simulink model "case_study_3"  (R2013a)
settings: Solver=ode45  SolverMode=SingleTasking  StartTime=0.0  StopTime=0.1  FixedStep=0.0001  RelTol=1e-2
undefined symbols (not defined in the file): f, ids, iqs, is, Ld, LL, Lq, P, RL, Rs, w
libraries: powerlib x34, simulink x12
settings Model: Creator=Asim Khan  LastModifiedBy=Sony
settings DataIOCC: SignalLoggingSaveFormat=ModelDataLogs
settings OptimizationCC: BlockReduction=off  BooleanDataType=off
settings DebuggingCC: SaveWithParameterizedLinksMsg=none  SignalResolutionControl=TryResolveAllWithWarning  SolverPrmCheckMsg=none  MultiTaskDSMMsg=warning  MultiTaskCondExecSysMsg=none  StrictBusMsg=None
settings HardwareCC: TargetUnknown=on
settings RTWCC: IncludeERTFirstTime=on

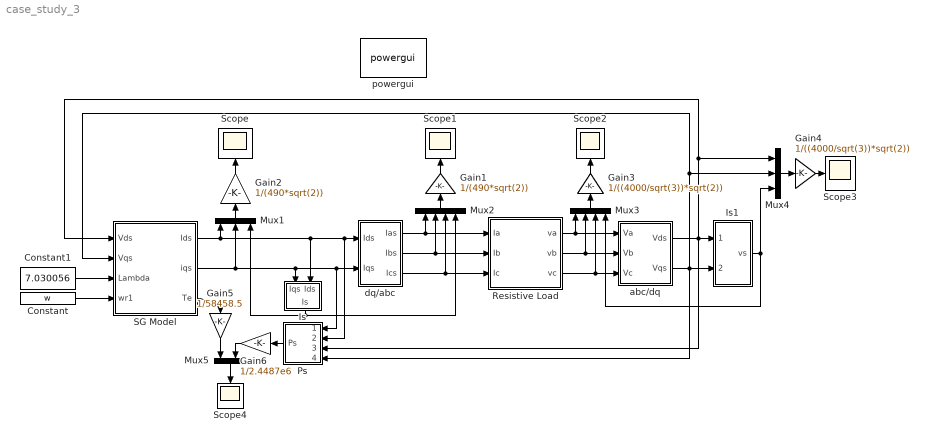
== system case_study_3 ==
  Constant : Constant  Value=w
  Constant1 : Constant  Value=7.030056
  Gain1 : Gain  Gain=1/(490*sqrt(2))
  Gain2 : Gain  Gain=1/(490*sqrt(2))
  Gain3 : Gain  Gain=1/((4000/sqrt(3))*sqrt(2))
  Gain4 : Gain  Gain=1/((4000/sqrt(3))*sqrt(2))
  Gain5 : Gain  Gain=1/58458.5
  Gain6 : Gain  Gain=1/2.4487e6
  Is : Subsystem
  Is1 : Subsystem
  Mux1 : Mux  Inputs=3
  Mux2 : Mux
  Mux3 : Mux
  Mux4 : Mux  Inputs=3
  Mux5 : Mux  Inputs=2
  Ps : Subsystem
  Resistive Load : Subsystem
  SG Model : Subsystem
  Scope{,1..4} (5 alike) : Scope
      Scope settings: YMin=0  YMax=1
      Scope1 settings: YMin=-0.8  YMax=0.8
      Scope4 settings: YMin=-20  YMax=20
  abc/dq : Subsystem
  "dq/abc " : Subsystem
  powergui : powerlib/powergui  Priority=1  SimulationMode=Continuous  SolverType=Tustin  SampleTime=50e-6  frequency=60  SPID=on  DisableSnubberDevices=off  DisableRonSwitches=on  DisableVfSwitches=on  SwTol=0  Interpol=off  DisplayEquations=off  frequencyindice=0  Pbase=100e6  ErrMax=1e-4  Iterations=50  UnitsV=kV  UnitsW=MW  FunctionMessages=off  echomessages=off  HookPort=off  EnableUseOfTLC=off  x0status=steady  RestoreLinks=warning  ResistiveCurrentMeasurement=off  Frange=[0:2:500]  Ylog=off  Xlog=on  ShowGrid=off  save=off  variable=ZData  ZoomFFT=off  StartTime=0.0  cycles=1  DisplayStyle=1  fundamental=60  FreqAxis=off  MaxFrequency=1000  frequencyindicesteady=1  RmsSteady=1  display=off  Ts=0  methode=off
  wires:
  SG Model/2(iqs) -> "dq/abc "/2(Iqs), Ps/1(Iqs), Is/1(Iqs), Mux1/2
  Resistive Load/1(va) -> abc/dq/1(Va), Mux3/1
  Resistive Load/2(vb) -> Mux3/2, abc/dq/2(Vb)
  Resistive Load/3(vc) -> abc/dq/3(Vc), Mux3/3
  Constant1/1 -> SG Model/3(Lambda)
  "dq/abc "/1(Ias) -> Resistive Load/1(Ia), Mux2/1
  "dq/abc "/2(Ibs) -> Resistive Load/2(Ib), Mux2/2
  "dq/abc "/3("Ics ") -> Resistive Load/3(Ic), Mux2/3
  abc/dq/1(Vds) -> Ps/3(vds), SG Model/1(Vds), Mux4/1, Is1/1(vds)
  SG Model/1(Ids) -> "dq/abc "/1(Ids), Ps/2(Ids), Is/2(Ids), Mux1/1
  Constant/1 -> SG Model/4(wr1)
  Mux5/1 -> Scope4/1
  Mux1/1 -> Gain2/1
  Gain2/1 -> Scope/1
  Mux2/1 -> Gain1/1
  Gain1/1 -> Scope1/1
  Mux3/1 -> Gain3/1
  Gain3/1 -> Scope2/1
  Mux4/1 -> Gain4/1
  Gain4/1 -> Scope3/1
  Is/1(Is) -> Mux2/4, Mux1/3
  abc/dq/2(Vqs) -> Ps/4(vqs), Is1/2(vqs), SG Model/2(Vqs), Mux4/2
  SG Model/3(Te) -> Gain5/1
  Gain5/1 -> Mux5/1
  Ps/1(Ps) -> Gain6/1
  Gain6/1 -> Mux5/2
  Is1/1(vs) -> Mux3/4, Mux4/3

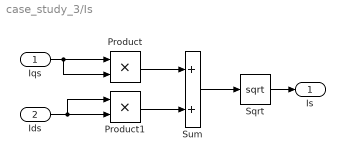
== system case_study_3/Is ==
  Iqs : Inport
  Ids : Inport  Port=2
  Product : Product
  Product1 : Product
  Sqrt : Sqrt  SaturateOnIntegerOverflow=on
  Sum : Sum
  Is : Outport
  wires:
  Iqs/1 -> Product/2, Product/1
  Ids/1 -> Product1/2, Product1/1
  Product/1 -> Sum/1
  Product1/1 -> Sum/2
  Sum/1 -> Sqrt/1
  Sqrt/1 -> Is/1

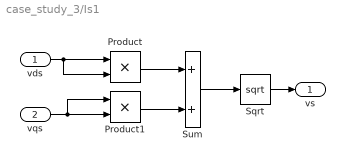
== system case_study_3/Is1 ==
  vds : Inport
  vqs : Inport  Port=2
  Product : Product
  Product1 : Product
  Sqrt : Sqrt  SaturateOnIntegerOverflow=on
  Sum : Sum
  vs : Outport
  wires:
  vds/1 -> Product/2, Product/1
  vqs/1 -> Product1/2, Product1/1
  Product/1 -> Sum/1
  Product1/1 -> Sum/2
  Sum/1 -> Sqrt/1
  Sqrt/1 -> vs/1

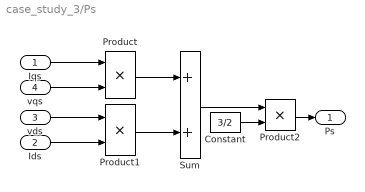
== system case_study_3/Ps ==
  Iqs : Inport
  Ids : Inport  Port=2
  vds : Inport  Port=3
  vqs : Inport  Port=4
  Constant : Constant  Value=3/2
  Product : Product
  Product1 : Product
  Product2 : Product
  Sum : Sum
  Ps : Outport
  wires:
  Iqs/1 -> Product/1
  Ids/1 -> Product1/2
  Product/1 -> Sum/1
  Product1/1 -> Sum/2
  Sum/1 -> Product2/1
  Constant/1 -> Product2/2
  vqs/1 -> Product/2
  vds/1 -> Product1/1
  Product2/1 -> Ps/1

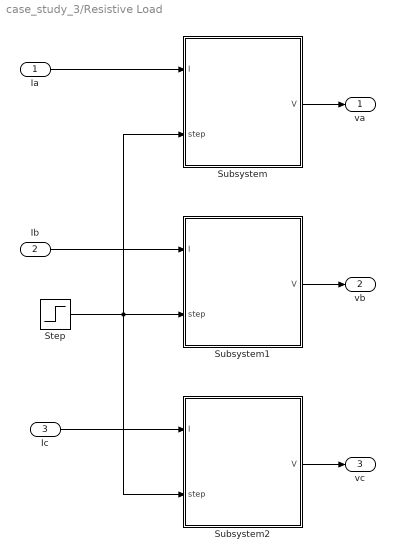
== system case_study_3/Resistive Load ==
  Ia : Inport
  Ib : Inport  Port=2
  Ic : Inport  Port=3
  Step : Step  Time=0.05  SampleTime=0
  Subsystem : Subsystem
  Subsystem1 : Subsystem
  Subsystem2 : Subsystem
  va : Outport
  vb : Outport  Port=2
  vc : Outport  Port=3
  wires:
  Step/1 -> Subsystem2/2(step), Subsystem1/2(step), Subsystem/2(step)
  Ia/1 -> Subsystem/1(I)
  Subsystem/1(V) -> va/1
  Subsystem1/1(V) -> vb/1
  Ib/1 -> Subsystem1/1(I)
  Ic/1 -> Subsystem2/1(I)
  Subsystem2/1(V) -> vc/1

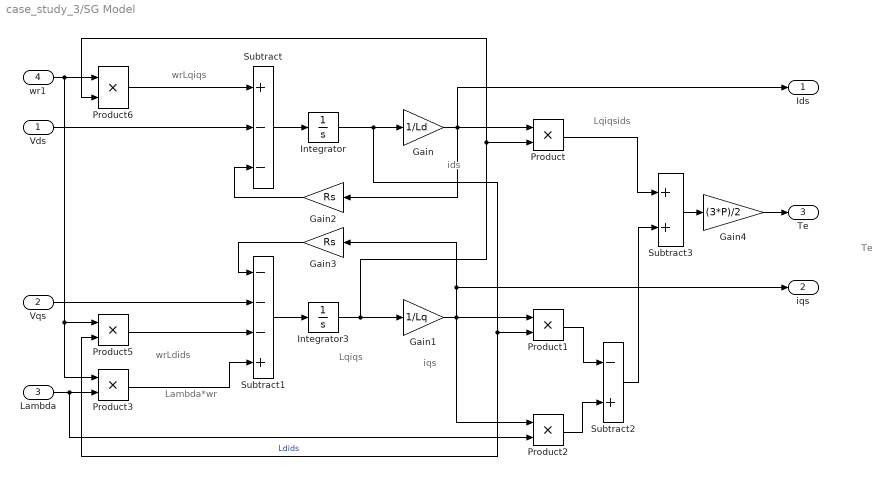
== system case_study_3/SG Model ==
  note: Lqiqsids
  note: iqs
  note: Te
  note: Lqiqs
  note: wrLqiqs
  note: wrLdids
  note: Lambda*wr
  note: ids
  Vds : Inport
  Vqs : Inport  Port=2
  Lambda : Inport  Port=3
  wr1 : Inport  Port=4
  Gain : Gain  Gain=1/Ld
  Gain1 : Gain  Gain=1/Lq
  Gain2 : Gain  Gain=Rs
  Gain3 : Gain  Gain=Rs
  Gain4 : Gain  Gain=(3*P)/2
  Integrator : Integrator  InitialCondition=ids*Ld
  Integrator3 : Integrator  InitialCondition=iqs*Lq
  Product{,1..3,5..6} (6 alike) : Product
  Subtract : Sum  Inputs=+--
  Subtract1 : Sum  Inputs=---+
  Subtract2 : Sum  Inputs=-+
  Subtract3 : Sum
  Ids : Outport
  iqs : Outport  Port=2
  Te : Outport  Port=3
  wires:
  Subtract/1 -> Integrator/1
  Subtract1/1 -> Integrator3/1
  Subtract3/1 -> Gain4/1
  Gain2/1 -> Subtract/3
  Gain3/1 -> Subtract1/1
  Integrator/1 -> Product1/2, Product5/2, Gain/1  "Ldids"
  Gain/1 -> Gain2/1, Product/1, Ids/1
  Gain1/1 -> Gain3/1, iqs/1, Product1/1, Product2/1
  Lambda/1 -> Product2/2, Product3/2
  Product/1 -> Subtract3/1
  Product1/1 -> Subtract2/1
  Product2/1 -> Subtract2/2
  Subtract2/1 -> Subtract3/2
  Gain4/1 -> Te/1
  Integrator3/1 -> Product6/2, Product/2, Gain1/1
  Vqs/1 -> Subtract1/2
  Vds/1 -> Subtract/2
  wr1/1 -> Product6/1, Product5/1, Product3/1
  Product6/1 -> Subtract/1
  Product5/1 -> Subtract1/3
  Product3/1 -> Subtract1/4

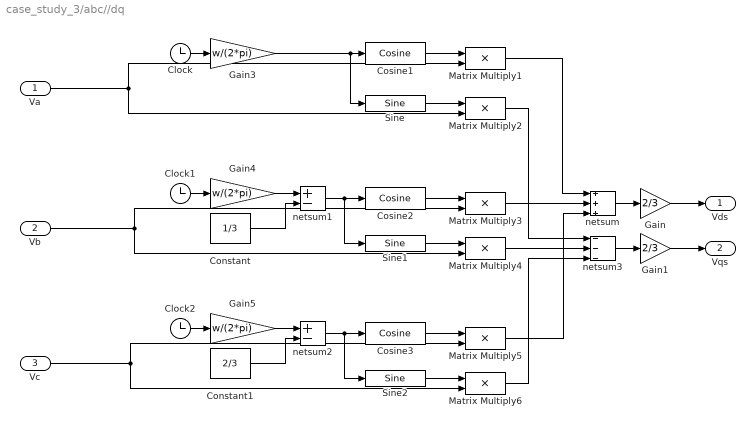
== system case_study_3/abc//dq ==
  Va : Inport
  Vb : Inport  Port=2
  Vc : Inport  Port=3
  Clock : Clock
  Clock1 : Clock
  Clock2 : Clock
  Constant : Constant  Value=1/3
  Constant1 : Constant  Value=2/3
  Cosine1 : simulink/Lookup Tables/Cosine  Formula=cos(2*pi*u)  NumDataPoints=(2^5)+1  OutputWordLength=16
  Cosine2 : simulink/Lookup Tables/Cosine  Formula=cos(2*pi*u)  NumDataPoints=(2^5)+1  OutputWordLength=16
  Cosine3 : simulink/Lookup Tables/Cosine  Formula=cos(2*pi*u)  NumDataPoints=(2^5)+1  OutputWordLength=16
  Gain : Gain  Gain=2/3
  Gain1 : Gain  Gain=2/3
  Gain3 : Gain  Gain=w/(2*pi)
  Gain4 : Gain  Gain=w/(2*pi)
  Gain5 : Gain  Gain=w/(2*pi)
  Matrix Multiply{1..6} (6 alike) : Product
  Sine : simulink/Lookup Tables/Sine  Formula=sin(2*pi*u)  NumDataPoints=(2^5)+1  OutputWordLength=16
  Sine1 : simulink/Lookup Tables/Sine  Formula=sin(2*pi*u)  NumDataPoints=(2^5)+1  OutputWordLength=16
  Sine2 : simulink/Lookup Tables/Sine  Formula=sin(2*pi*u)  NumDataPoints=(2^5)+1  OutputWordLength=16
  netsum : Sum  Inputs=+++  SaturateOnIntegerOverflow=on  InputSameDT=on  OutDataTypeStr=Inherit: Same as first input
  netsum1 : Sum  Inputs=+-  SaturateOnIntegerOverflow=on  InputSameDT=on  OutDataTypeStr=Inherit: Same as first input
  netsum2 : Sum  Inputs=+-  SaturateOnIntegerOverflow=on  InputSameDT=on  OutDataTypeStr=Inherit: Same as first input
  netsum3 : Sum  Inputs=---  SaturateOnIntegerOverflow=on  InputSameDT=on  OutDataTypeStr=Inherit: Same as first input
  Vds : Outport
  Vqs : Outport  Port=2
  wires:
  Cosine1/1 -> Matrix Multiply1/1
  Clock/1 -> Gain3/1
  Gain3/1 -> Sine/1, Cosine1/1
  Sine/1 -> Matrix Multiply2/1
  Cosine2/1 -> Matrix Multiply3/1
  Clock1/1 -> Gain4/1
  Sine1/1 -> Matrix Multiply4/1
  Gain4/1 -> netsum1/1
  netsum1/1 -> Sine1/1, Cosine2/1
  Constant/1 -> netsum1/2
  Cosine3/1 -> Matrix Multiply5/1
  Clock2/1 -> Gain5/1
  Sine2/1 -> Matrix Multiply6/1
  Gain5/1 -> netsum2/1
  netsum2/1 -> Sine2/1, Cosine3/1
  Constant1/1 -> netsum2/2
  Gain1/1 -> Vqs/1
  Gain/1 -> Vds/1
  Va/1 -> Matrix Multiply2/2, Matrix Multiply1/2
  Vb/1 -> Matrix Multiply4/2, Matrix Multiply3/2
  Vc/1 -> Matrix Multiply6/2, Matrix Multiply5/2
  Matrix Multiply1/1 -> netsum/1
  Matrix Multiply3/1 -> netsum/2
  Matrix Multiply5/1 -> netsum/3
  netsum/1 -> Gain/1
  netsum3/1 -> Gain1/1
  Matrix Multiply2/1 -> netsum3/1
  Matrix Multiply4/1 -> netsum3/2
  Matrix Multiply6/1 -> netsum3/3

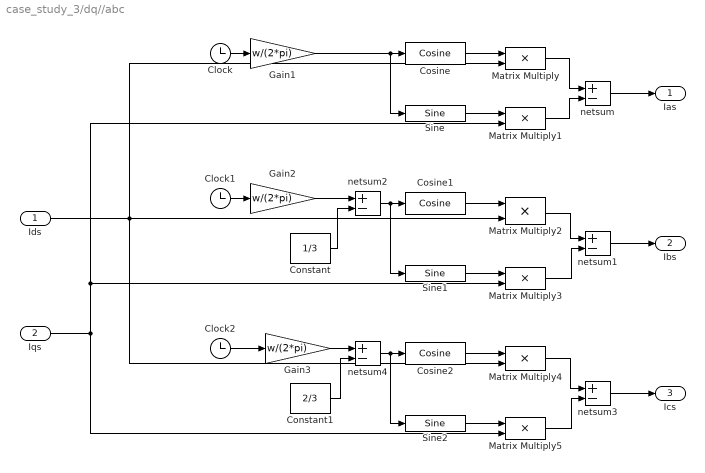
== system case_study_3/dq//abc  ==
  Ids : Inport
  Iqs : Inport  Port=2
  Clock : Clock
  Clock1 : Clock
  Clock2 : Clock
  Constant : Constant  Value=1/3
  Constant1 : Constant  Value=2/3
  Cosine : simulink/Lookup Tables/Cosine  Formula=cos(2*pi*u)  NumDataPoints=(2^5)+1  OutputWordLength=16
  Cosine1 : simulink/Lookup Tables/Cosine  Formula=cos(2*pi*u)  NumDataPoints=(2^5)+1  OutputWordLength=16
  Cosine2 : simulink/Lookup Tables/Cosine  Formula=cos(2*pi*u)  NumDataPoints=(2^5)+1  OutputWordLength=16
  Gain1 : Gain  Gain=w/(2*pi)
  Gain2 : Gain  Gain=w/(2*pi)
  Gain3 : Gain  Gain=w/(2*pi)
  Matrix Multiply{,1..5} (6 alike) : Product
  Sine : simulink/Lookup Tables/Sine  Formula=sin(2*pi*u)  NumDataPoints=(2^5)+1  OutputWordLength=16
  Sine1 : simulink/Lookup Tables/Sine  Formula=sin(2*pi*u)  NumDataPoints=(2^5)+1  OutputWordLength=16
  Sine2 : simulink/Lookup Tables/Sine  Formula=sin(2*pi*u)  NumDataPoints=(2^5)+1  OutputWordLength=16
  netsum{,1..4} (5 alike) : Sum  Inputs=+-  SaturateOnIntegerOverflow=on  InputSameDT=on  OutDataTypeStr=Inherit: Same as first input
  Ias : Outport
  Ibs : Outport  Port=2
  "Ics " : Outport  Port=3
  wires:
  Clock/1 -> Gain1/1
  Gain1/1 -> Sine/1, Cosine/1
  Matrix Multiply/1 -> netsum/1
  Matrix Multiply1/1 -> netsum/2
  netsum/1 -> Ias/1
  Clock1/1 -> Gain2/1
  Sine1/1 -> Matrix Multiply3/1
  Matrix Multiply2/1 -> netsum1/1
  Matrix Multiply3/1 -> netsum1/2
  netsum1/1 -> Ibs/1
  Gain2/1 -> netsum2/1
  netsum2/1 -> Sine1/1, Cosine1/1
  Constant/1 -> netsum2/2
  Clock2/1 -> Gain3/1
  Sine2/1 -> Matrix Multiply5/1
  Matrix Multiply4/1 -> netsum3/1
  Matrix Multiply5/1 -> netsum3/2
  netsum3/1 -> "Ics "/1
  Gain3/1 -> netsum4/1
  netsum4/1 -> Sine2/1, Cosine2/1
  Constant1/1 -> netsum4/2
  Ids/1 -> Matrix Multiply4/2, Matrix Multiply/2, Matrix Multiply2/2
  Iqs/1 -> Matrix Multiply1/2, Matrix Multiply3/2, Matrix Multiply5/2
  Cosine/1 -> Matrix Multiply/1
  Sine/1 -> Matrix Multiply1/1
  Cosine1/1 -> Matrix Multiply2/1
  Cosine2/1 -> Matrix Multiply4/1

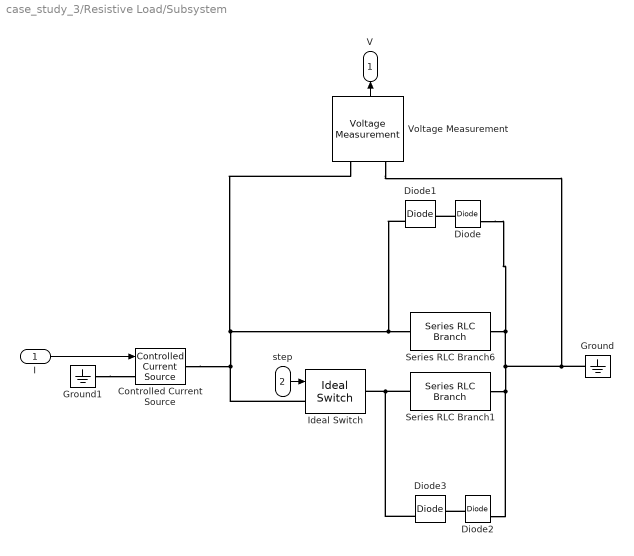
== system case_study_3/Resistive Load/Subsystem ==
  I : Inport
  step : Inport  Port=2
  Controlled Current Source : powerlib/Electrical Sources/Controlled Current Source  Initialize=off  Source_Type=AC  Amplitude=is  Phase=90  Frequency=f  Measurements=None
  Diode{,1..3} (4 alike) : powerlib/Power Electronics/Diode  Ron=0.001  Lon=0  Vf=0.8  IC=0  UseSnubber=off  Rs=Rsnubber  Cs=inf  Measurements=on
  Ground : powerlib/Elements/Ground  LConnTagsString=a
  Ground1 : powerlib/Elements/Ground  LConnTagsString=a
  Ideal Switch : powerlib/Power Electronics/Ideal Switch  Ron=0.001  Lon=0  IC=0  Rs=inf  Cs=inf  Measurements=off
  Series RLC Branch1 : powerlib/Elements/Series RLC Branch  LConnTagsString=__new0  RConnTagsString=__new0  BranchType=RL  Resistance=RL  Inductance=LL  SetiL0=on  InitialCurrent=is  Capacitance=0  Setx0=off  InitialVoltage=0  Measurements=None
  Series RLC Branch6 : powerlib/Elements/Series RLC Branch  LConnTagsString=__new0  RConnTagsString=__new0  BranchType=RL  Resistance=RL  Inductance=LL  SetiL0=on  InitialCurrent=is  Capacitance=0  Setx0=off  InitialVoltage=0  Measurements=None
  Voltage Measurement : powerlib/Measurements/Voltage Measurement  PhasorSimulation=off  OutputType=Complex  PSBequivalent=0
  V : Outport
  wires:
  Voltage Measurement/1 -> V/1
  I/1 -> Controlled Current Source/1
  step/1 -> Ideal Switch/1
  connections:
  Series RLC Branch1/LConn1 -- Diode3/RConn1 -- Ideal Switch/RConn1
  Controlled Current Source/RConn1 -- Ideal Switch/LConn1 -- Voltage Measurement/LConn1 -- Diode1/RConn1 -- Series RLC Branch6/LConn1
  Voltage Measurement/LConn2 -- Ground/LConn1 -- Diode/RConn1 -- Series RLC Branch6/RConn1 -- Diode2/RConn1 -- Series RLC Branch1/RConn1
  Ground1/LConn1 -- Controlled Current Source/LConn1
  Diode/LConn1 -- Diode1/LConn1
  Diode2/LConn1 -- Diode3/LConn1

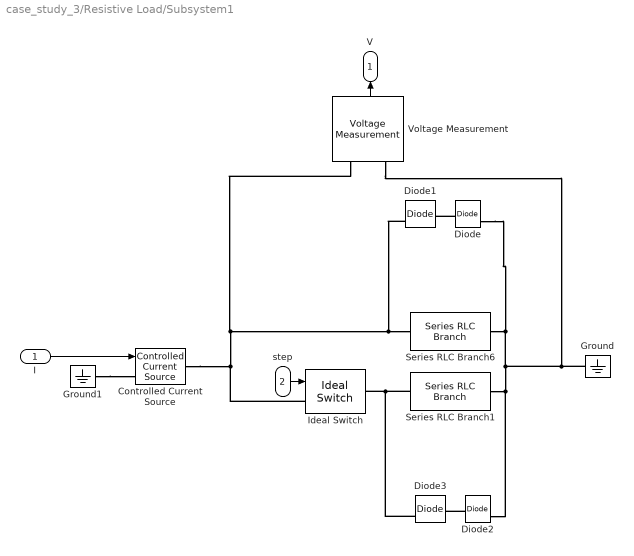
== system case_study_3/Resistive Load/Subsystem1 ==
  I : Inport
  step : Inport  Port=2
  Controlled Current Source : powerlib/Electrical Sources/Controlled Current Source  Initialize=off  Source_Type=AC  Amplitude=is  Phase=90  Frequency=f  Measurements=None
  Diode{,1..3} (4 alike) : powerlib/Power Electronics/Diode  Ron=0.001  Lon=0  Vf=0.8  IC=0  UseSnubber=off  Rs=Rsnubber  Cs=inf  Measurements=on
  Ground : powerlib/Elements/Ground  LConnTagsString=a
  Ground1 : powerlib/Elements/Ground  LConnTagsString=a
  Ideal Switch : powerlib/Power Electronics/Ideal Switch  Ron=0.001  Lon=0  IC=0  Rs=inf  Cs=inf  Measurements=off
  Series RLC Branch1 : powerlib/Elements/Series RLC Branch  LConnTagsString=__new0  RConnTagsString=__new0  BranchType=RL  Resistance=RL  Inductance=LL  SetiL0=on  InitialCurrent=is  Capacitance=0  Setx0=off  InitialVoltage=0  Measurements=None
  Series RLC Branch6 : powerlib/Elements/Series RLC Branch  LConnTagsString=__new0  RConnTagsString=__new0  BranchType=RL  Resistance=RL  Inductance=LL  SetiL0=on  InitialCurrent=is  Capacitance=0  Setx0=off  InitialVoltage=0  Measurements=None
  Voltage Measurement : powerlib/Measurements/Voltage Measurement  PhasorSimulation=off  OutputType=Complex  PSBequivalent=0
  V : Outport
  wires:
  Voltage Measurement/1 -> V/1
  I/1 -> Controlled Current Source/1
  step/1 -> Ideal Switch/1
  connections:
  Diode3/RConn1 -- Series RLC Branch1/LConn1 -- Ideal Switch/RConn1
  Diode1/RConn1 -- Controlled Current Source/RConn1 -- Ideal Switch/LConn1 -- Voltage Measurement/LConn1 -- Series RLC Branch6/LConn1
  Diode2/RConn1 -- Voltage Measurement/LConn2 -- Ground/LConn1 -- Diode/RConn1 -- Series RLC Branch6/RConn1 -- Series RLC Branch1/RConn1
  Ground1/LConn1 -- Controlled Current Source/LConn1
  Diode/LConn1 -- Diode1/LConn1
  Diode2/LConn1 -- Diode3/LConn1

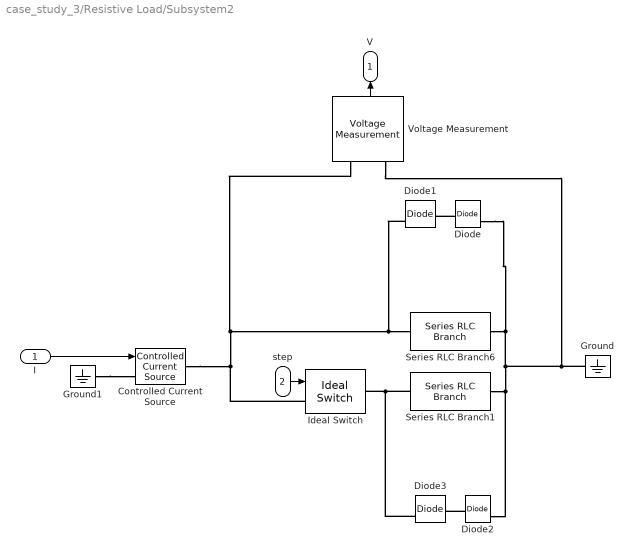
== system case_study_3/Resistive Load/Subsystem2 ==
  I : Inport
  step : Inport  Port=2
  Controlled Current Source : powerlib/Electrical Sources/Controlled Current Source  Initialize=off  Source_Type=AC  Amplitude=is  Phase=90  Frequency=f  Measurements=None
  Diode{,1..3} (4 alike) : powerlib/Power Electronics/Diode  Ron=0.001  Lon=0  Vf=0.8  IC=0  UseSnubber=off  Rs=Rsnubber  Cs=inf  Measurements=on
  Ground : powerlib/Elements/Ground  LConnTagsString=a
  Ground1 : powerlib/Elements/Ground  LConnTagsString=a
  Ideal Switch : powerlib/Power Electronics/Ideal Switch  Ron=0.001  Lon=0  IC=0  Rs=inf  Cs=inf  Measurements=off
  Series RLC Branch1 : powerlib/Elements/Series RLC Branch  LConnTagsString=__new0  RConnTagsString=__new0  BranchType=RL  Resistance=RL  Inductance=LL  SetiL0=on  InitialCurrent=is  Capacitance=0  Setx0=off  InitialVoltage=0  Measurements=None
  Series RLC Branch6 : powerlib/Elements/Series RLC Branch  LConnTagsString=__new0  RConnTagsString=__new0  BranchType=RL  Resistance=RL  Inductance=LL  SetiL0=on  InitialCurrent=is  Capacitance=0  Setx0=off  InitialVoltage=0  Measurements=None
  Voltage Measurement : powerlib/Measurements/Voltage Measurement  PhasorSimulation=off  OutputType=Complex  PSBequivalent=0
  V : Outport
  wires:
  Voltage Measurement/1 -> V/1
  I/1 -> Controlled Current Source/1
  step/1 -> Ideal Switch/1
  connections:
  Diode3/RConn1 -- Series RLC Branch1/LConn1 -- Ideal Switch/RConn1
  Diode1/RConn1 -- Controlled Current Source/RConn1 -- Ideal Switch/LConn1 -- Voltage Measurement/LConn1 -- Series RLC Branch6/LConn1
  Diode2/RConn1 -- Voltage Measurement/LConn2 -- Ground/LConn1 -- Diode/RConn1 -- Series RLC Branch6/RConn1 -- Series RLC Branch1/RConn1
  Ground1/LConn1 -- Controlled Current Source/LConn1
  Diode/LConn1 -- Diode1/LConn1
  Diode2/LConn1 -- Diode3/LConn1
